simulink library "INT_RngMod_TrqCalc"  (R2016b)
settings: Solver=VariableStepAuto  StartTime=0.0  StopTime=10.0  RelTol=1e-3
settings Model: Creator=Administrator  LastModifiedBy=Administrator

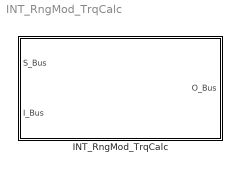
== system INT_RngMod_TrqCalc ==
  INT_RngMod_TrqCalc : Subsystem

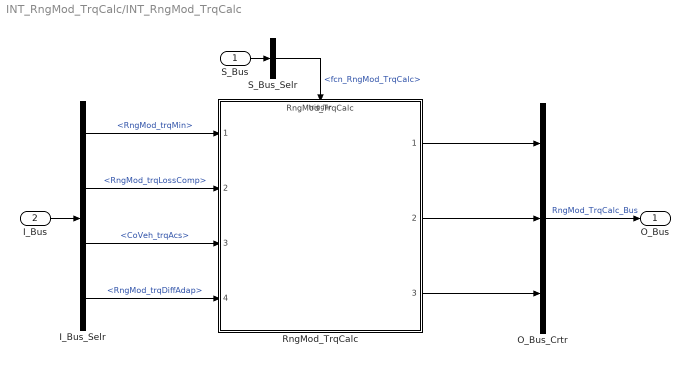
== system INT_RngMod_TrqCalc/INT_RngMod_TrqCalc ==
  S_Bus : Inport
  I_Bus : Inport  Port=2
  I_Bus_Selr : BusSelector  OutputSignals=RngMod_trqMin,RngMod_trqLossComp,CoVeh_trqAcs,RngMod_trqDiffAdap
  O_Bus_Crtr : BusCreator  Inputs=3
  RngMod_TrqCalc : ModelReference  ModelNameDialog=RngMod_TrqCalc  SimulationMode=Normal  ModelReferenceVersion=1.8  TriggerPortName=function  TriggerPortTriggerType=function-call  TriggerPortStatesWhenEnabling=held
  S_Bus_Selr : BusSelector  OutputSignals=fcn_RngMod_TrqCalc
  O_Bus : Outport
  wires:
  S_Bus_Selr/1 -> RngMod_TrqCalc/Trigger  "<fcn_RngMod_TrqCalc>"
  S_Bus/1 -> S_Bus_Selr/1
  I_Bus/1 -> I_Bus_Selr/1
  I_Bus_Selr/1 -> RngMod_TrqCalc/1  "<RngMod_trqMin>"
  I_Bus_Selr/2 -> RngMod_TrqCalc/2  "<RngMod_trqLossComp>"
  I_Bus_Selr/3 -> RngMod_TrqCalc/3  "<CoVeh_trqAcs>"
  I_Bus_Selr/4 -> RngMod_TrqCalc/4  "<RngMod_trqDiffAdap>"
  O_Bus_Crtr/1 -> O_Bus/1  "RngMod_TrqCalc_Bus"
  RngMod_TrqCalc/1 -> O_Bus_Crtr/1
  RngMod_TrqCalc/2 -> O_Bus_Crtr/2
  RngMod_TrqCalc/3 -> O_Bus_Crtr/3
